simulink model "MPC_X4Constraints"  (R2022a)
settings: Solver=FixedStepDiscrete  StartTime=0.0  StopTime=T_sim  FixedStep=Ts  RelTol=1e-3  EnableMultiTasking=on
undefined symbols (not defined in the file or in its folder): C_states, D_states, MPCwithX2Constraints, MPCwithX4Constraints, N, over_shot_constraint, P_MPC, Q_MPC, R_MPC, sat_max, sat_min, sysd, Ts, x0, x2_max, x2_min, x_ref
settings Model: Creator=Mirko  LastModifiedBy=david
settings SolverCC: AlgebraicLoopSolver=TrustRegion
settings DataIOCC: LimitDataPoints=on  SaveFormat=Array  SignalLoggingSaveFormat=ModelDataLogs  ReturnWorkspaceOutputs=off
settings OptimizationCC: ExpressionDepthLimit=2147483647  LifeSpan=inf
settings DebuggingCC: UnderspecifiedInitializationDetection=Classic  MergeDetectMultiDrivingBlocksExec=none  FcnCallInpInsideContextMsg=warning  UnconnectedInputMsg=warning  UnconnectedOutputMsg=warning  UnconnectedLineMsg=warning  StateNameClashWarn=warning  SFUnexpectedBacktrackingDiag=warning  SFNoUnconditionalDefaultTransitionDiag=warning  SFExecutionAtInitializationDiag=none  SFMachineParentedDataDiag=warning  ArithmeticOperatorsInVariantConditions=warning
settings HardwareCC: ProdBitPerPointer=32  ProdBitPerSizeT=32  ProdBitPerPtrDiffT=32  ProdLargestAtomicFloat=None  ProdIntDivRoundTo=Undefined  ProdEndianess=Unspecified  ProdWordSize=32  ProdHWDeviceType=32-bit Generic
settings ModelReferenceCC: PropagateSignalLabelsOutOfModel=off
settings SFSimCC: SimUseLocalCustomCode=off  CustomCodeUndefinedFunction=UseInterfaceOnly
settings RTWCC: RTWUseLocalCustomCode=off  DLArmComputeVersion=19.05
settings CodeAppCC: StateflowObjectComments=on
settings GRTTargetCC: TargetLangStandard=C89/C90 (ANSI)
settings ConfigComp: CovMetricSettings=dw  CovSaveCumulativeToWorkspaceVar=on  CovSaveSingleToWorkspaceVar=on  CovExternalEMLEnable=off  CovSFcnEnable=off

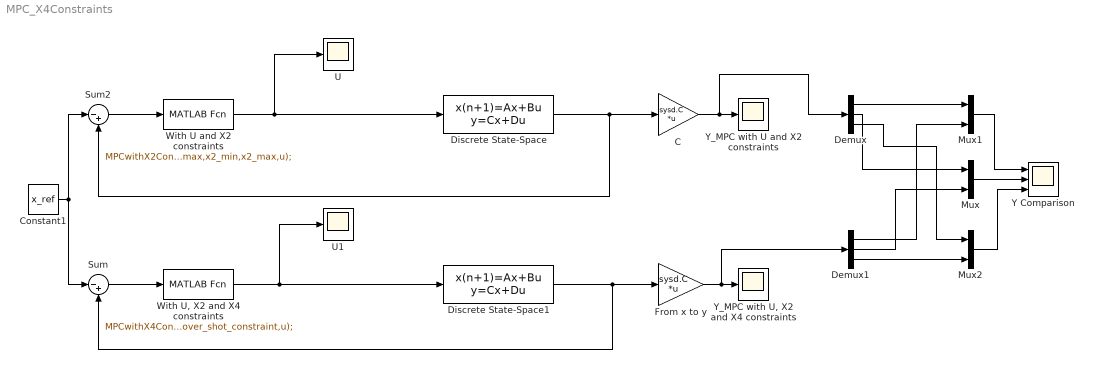
== system MPC_X4Constraints ==
  C : Gain  Gain=sysd.C  Multiplication=Matrix(K*u)
  Constant1 : Constant  Value=x_ref
  Demux : Demux  Outputs=3
  Demux1 : Demux  Outputs=3
  Discrete State-Space : DiscreteStateSpace  A=sysd.A  B=sysd.B  C=C_states  D=D_states  InitialCondition=x0  SampleTime=Ts
  Discrete State-Space1 : DiscreteStateSpace  A=sysd.A  B=sysd.B  C=C_states  D=D_states  InitialCondition=x0  SampleTime=Ts
  From x to y : Gain  Gain=sysd.C  Multiplication=Matrix(K*u)
  Mux : Mux  Inputs=2
  Mux1 : Mux  Inputs=2
  Mux2 : Mux  Inputs=2
  Sum : Sum  Inputs=|-+
  Sum2 : Sum  Inputs=|-+
  U : Scope
  U1 : Scope
  With U and X2 constraints : MATLABFcn  MATLABFcn=MPCwithX2Constraints(sysd.A,sysd.B,Q_MPC,R_MPC,P_MPC,N,sat_min,sat_max,x2_min,x2_max,u);  OutputDimensions=1
  "With U, X2 and X4 constraints" : MATLABFcn  MATLABFcn=MPCwithX4Constraints(sysd.A,sysd.B,Q_MPC,R_MPC,P_MPC,N,sat_min,sat_max,x2_min,x2_max,sign(x0(4)),over_shot_constraint,u);  OutputDimensions=1
  Y Comparison : Scope  NumInputPorts=3
  Y_MPC with U and X2 constraints : Scope
  "Y_MPC with U, X2 and X4 constraints" : Scope
  wires:
  Discrete State-Space1/1 -> Sum/2, From x to y/1
  Sum/1 -> "With U, X2 and X4 constraints"/1
  From x to y/1 -> "Y_MPC with U, X2 and X4 constraints"/1, Demux1/1
  "With U, X2 and X4 constraints"/1 -> Discrete State-Space1/1, U1/1
  With U and X2 constraints/1 -> Discrete State-Space/1, U/1
  Sum2/1 -> With U and X2 constraints/1
  Discrete State-Space/1 -> C/1, Sum2/2
  Demux/1 -> Mux1/1
  Mux1/1 -> Y Comparison/1
  Demux1/1 -> Mux1/2
  Demux/2 -> Mux/1
  Demux1/2 -> Mux/2
  Demux1/3 -> Mux2/2
  Demux/3 -> Mux2/1
  Mux2/1 -> Y Comparison/3
  Mux/1 -> Y Comparison/2
  C/1 -> Y_MPC with U and X2 constraints/1, Demux/1
  Constant1/1 -> Sum/1, Sum2/1
